simulink library "INT_ActMod_Q2Trq"  (R2016b)
settings: Solver=VariableStepAuto  StartTime=0.0  StopTime=10.0  RelTol=1e-3
settings Model: Creator=Administrator  LastModifiedBy=Administrator

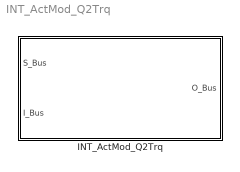
== system INT_ActMod_Q2Trq ==
  INT_ActMod_Q2Trq : Subsystem

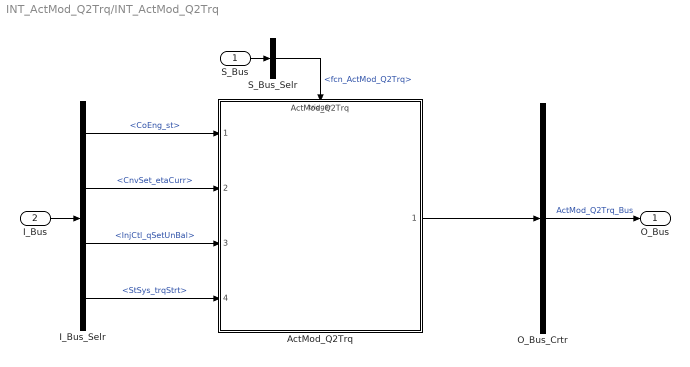
== system INT_ActMod_Q2Trq/INT_ActMod_Q2Trq ==
  S_Bus : Inport
  I_Bus : Inport  Port=2
  ActMod_Q2Trq : ModelReference  ModelNameDialog=ActMod_Q2Trq  SimulationMode=Normal  ModelReferenceVersion=1.2  TriggerPortName=function  TriggerPortTriggerType=function-call  TriggerPortStatesWhenEnabling=held
  I_Bus_Selr : BusSelector  OutputSignals=CoEng_st,CnvSet_etaCurr,InjCtl_qSetUnBal,StSys_trqStrt
  O_Bus_Crtr : BusCreator  Inputs=1
  S_Bus_Selr : BusSelector  OutputSignals=fcn_ActMod_Q2Trq
  O_Bus : Outport
  wires:
  S_Bus_Selr/1 -> ActMod_Q2Trq/Trigger  "<fcn_ActMod_Q2Trq>"
  S_Bus/1 -> S_Bus_Selr/1
  I_Bus/1 -> I_Bus_Selr/1
  I_Bus_Selr/1 -> ActMod_Q2Trq/1  "<CoEng_st>"
  I_Bus_Selr/2 -> ActMod_Q2Trq/2  "<CnvSet_etaCurr>"
  I_Bus_Selr/3 -> ActMod_Q2Trq/3  "<InjCtl_qSetUnBal>"
  I_Bus_Selr/4 -> ActMod_Q2Trq/4  "<StSys_trqStrt>"
  O_Bus_Crtr/1 -> O_Bus/1  "ActMod_Q2Trq_Bus"
  ActMod_Q2Trq/1 -> O_Bus_Crtr/1
